simulink model "pendulum"  (R2024b)
settings: Solver=VariableStepAuto  StartTime=0.0  StopTime=80.0  RelTol=1e-3
undefined symbols (not defined in the file): c, d, g, J, L, m
libraries: fuzblock x1, simulink_extras x1

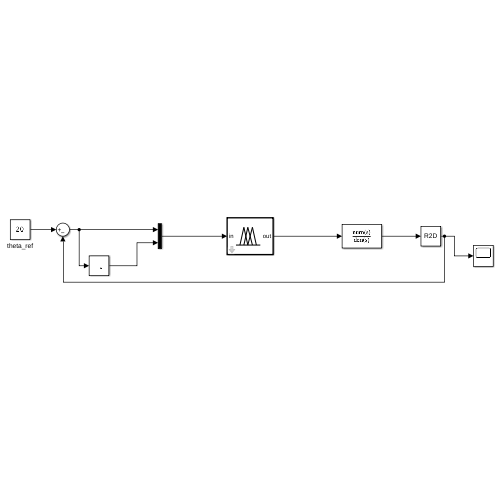
[thumbnail: Simulink's stored preview of the top-level diagram]
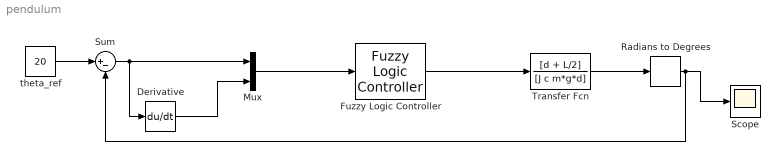
== system pendulum ==
  Derivative : Derivative
  Fuzzy Logic Controller : fuzblock/Fuzzy Logic  Controller  FIS=pendulum_fuzzy  OutputSampleNumber=101  DataType=double  FuzzifiedInputs=off  RuleFiringStrengths=off  RuleOutputs=off  AggregatedOutputs=off  SimulateUsing=Interpreted execution  OutOfRangeInputValueMessage=warning  NoRuleFiredMessage=warning  EmptyOutputFuzzySetMessage=warning
  Mux : Mux  Inputs=2
  Radians to Degrees : simulink_extras/Transformations/Radians to Degrees
  Scope : Scope
  Sum : Sum  Inputs=|+-
  Transfer Fcn : TransferFcn  Numerator=[d + L/2]  Denominator=[J c m*g*d]
  theta_ref : Constant  Value=20
  wires:
  theta_ref/1 -> Sum/1
  Derivative/1 -> Mux/2
  Sum/1 -> Derivative/1, Mux/1
  Mux/1 -> Fuzzy Logic Controller/1
  Fuzzy Logic Controller/1 -> Transfer Fcn/1
  Transfer Fcn/1 -> Radians to Degrees/1
  Radians to Degrees/1 -> Sum/2, Scope/1
